simulink library "lib_Convection_TubeBankZukauskas"  (R2015a)
settings: Solver=ode45  StartTime=0.0  StopTime=10.0  RelTol=1e-3
libraries: simulink x24, lib_GenTools_MinMax x1
settings Model: Creator=jlkratz  LastModifiedBy=jlkratz

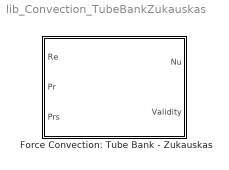
== system lib_Convection_TubeBankZukauskas ==
  Force Convection: Tube Bank - Zukauskas : Subsystem  mask(TSAT: Tube Bank - Zukauskas){N_M=20, StSLratio_M=4, AlignOrStag_M=on}
      mask prompts: N_M "N_M - Number of rows of tubes"; StSLratio_M "StSLratio_M - Ratio of distances between tubes in the transverse direction and flow direction (St/SL)"; AlignOrStag_M "AlignOrStag_M - Checked for aligned tubes and unchecked for staggered tubes"
      mask help:
      | This block estimates the average Nusselt number for an entire bank of cylinderical tubes using a correlation proposed by Zukauskas. The tube bank may consist of rows of tubes that are aligned with each other or staggered. The Reynolds number (Re) should be calculated based on the diameter of the largest cylinder in the bank. The properties of the fluid should be evaluated at the mean of the fluid inlet and outlet temperatures with the exception of Prs which is the Prantl number (Pr) evaluated using the temperature of the surface of the tubes. If the surface temperature of each tube differs then a rough approximation could be possible by using the average surface temperature of all the tubes. The correlation is best suited for banks with 20 or more rows of tubes but this implemenation does consider adjustments for banks with less than 20 rows. The correlation is subject to the following restricitons:
      |
      | 10 <= Re <= 2000000
      | 0.7 <= Pr <= 500
      |
      | For additional information see the block help menu.
      mask Help: web(which('Convection_TSAT_TubeBankZukauskus.html'),'-helpbrowser')
      mask DialogControl Container3 Prompt: Parameters

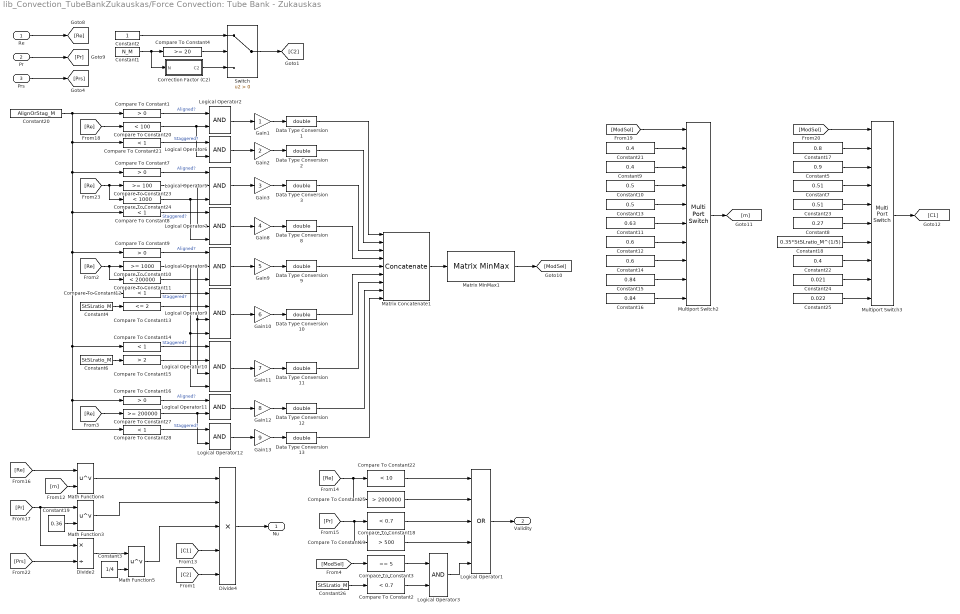
== system lib_Convection_TubeBankZukauskas/Force Convection: Tube Bank - Zukauskas ==
  Re : Inport
  Pr : Inport  Port=2
  Prs : Inport  Port=3
  Compare To Constant{1,7,9,16} (4 alike) : simulink/Logic and Bit Operations/Compare To Constant  relop=>  const=0  OutDataTypeStr=boolean
  Compare To Constant10 : simulink/Logic and Bit Operations/Compare To Constant  relop=>=  const=1000  OutDataTypeStr=boolean
  Compare To Constant11 : simulink/Logic and Bit Operations/Compare To Constant  relop=<  const=200000  OutDataTypeStr=boolean
  Compare To Constant{8,12,14,21,28} (5 alike) : simulink/Logic and Bit Operations/Compare To Constant  relop=<  const=1  OutDataTypeStr=boolean
  Compare To Constant13 : simulink/Logic and Bit Operations/Compare To Constant  relop=<=  const=2  OutDataTypeStr=boolean
  Compare To Constant15 : simulink/Logic and Bit Operations/Compare To Constant  relop=>  const=2  OutDataTypeStr=boolean
  Compare To Constant18 : simulink/Logic and Bit Operations/Compare To Constant  relop=<  const=0.7  OutDataTypeStr=boolean
  Compare To Constant19 : simulink/Logic and Bit Operations/Compare To Constant  relop=>  const=500  OutDataTypeStr=boolean
  Compare To Constant2 : simulink/Logic and Bit Operations/Compare To Constant  relop=<  const=0.7  OutDataTypeStr=boolean
  Compare To Constant20 : simulink/Logic and Bit Operations/Compare To Constant  relop=<  const=100  OutDataTypeStr=boolean
  Compare To Constant22 : simulink/Logic and Bit Operations/Compare To Constant  relop=<  const=10  OutDataTypeStr=boolean
  Compare To Constant23 : simulink/Logic and Bit Operations/Compare To Constant  relop=>=  const=100  OutDataTypeStr=boolean
  Compare To Constant24 : simulink/Logic and Bit Operations/Compare To Constant  relop=<  const=1000  OutDataTypeStr=boolean
  Compare To Constant25 : simulink/Logic and Bit Operations/Compare To Constant  relop=>  const=2000000  OutDataTypeStr=boolean
  Compare To Constant27 : simulink/Logic and Bit Operations/Compare To Constant  relop=>=  const=200000  OutDataTypeStr=boolean
  Compare To Constant3 : simulink/Logic and Bit Operations/Compare To Constant  relop===  const=5  OutDataTypeStr=boolean
  Compare To Constant4 : simulink/Logic and Bit Operations/Compare To Constant  relop=>=  const=20  OutDataTypeStr=boolean
  Constant1 : Constant  Value=N_M
  Constant10 : Constant  Value=0.5
  Constant11 : Constant  Value=0.63
  Constant12 : Constant  Value=0.6
  Constant13 : Constant  Value=0.5
  Constant14 : Constant  Value=0.6
  Constant15 : Constant  Value=0.84
  Constant16 : Constant  Value=0.84
  Constant17 : Constant  Value=0.8
  Constant18 : Constant  Value=0.35*StSLratio_M^(1/5)
  Constant19 : Constant  Value=0.36
  Constant2 : Constant
  Constant20 : Constant  Value=AlignOrStag_M
  Constant21 : Constant  Value=0.4
  Constant22 : Constant  Value=0.4
  Constant23 : Constant  Value=0.51
  Constant24 : Constant  Value=0.021
  Constant25 : Constant  Value=0.022
  Constant26 : Constant  Value=StSLratio_M
  Constant3 : Constant  Value=1/4
  Constant4 : Constant  Value=StSLratio_M
  Constant5 : Constant  Value=0.9
  Constant6 : Constant  Value=StSLratio_M
  Constant7 : Constant  Value=0.51
  Constant8 : Constant  Value=0.27
  Constant9 : Constant  Value=0.4
  Correction Factor (C2) : Subsystem
  Data Type Conversion{1..3,8..13} (9 alike) : DataTypeConversion  OutDataTypeStr=double
  Divide2 : Product  Inputs=*/
  Divide4 : Product  Inputs=*****
  Gain1 : Gain
  Gain10 : Gain  Gain=6
  Gain11 : Gain  Gain=7
  Gain12 : Gain  Gain=8
  Gain13 : Gain  Gain=9
  Gain2 : Gain  Gain=2
  Gain3 : Gain  Gain=3
  Gain8 : Gain  Gain=4
  Gain9 : Gain  Gain=5
  Logical Operator1 : Logic  Operator=OR  Inputs=5  AllPortsSameDT=off  OutDataTypeStr=boolean
  Logical Operator10 : Logic  Inputs=4  AllPortsSameDT=off  OutDataTypeStr=boolean
  Logical Operator{2..3,6,11..12} (5 alike) : Logic  AllPortsSameDT=off  OutDataTypeStr=boolean
  Logical Operator5 : Logic  Inputs=3  AllPortsSameDT=off  OutDataTypeStr=boolean
  Logical Operator7 : Logic  Inputs=3  AllPortsSameDT=off  OutDataTypeStr=boolean
  Logical Operator8 : Logic  Inputs=3  AllPortsSameDT=off  OutDataTypeStr=boolean
  Logical Operator9 : Logic  Inputs=4  AllPortsSameDT=off  OutDataTypeStr=boolean
  Math Function3 : Math  Operator=pow  SaturateOnIntegerOverflow=on
  Math Function4 : Math  Operator=pow  SaturateOnIntegerOverflow=on
  Math Function5 : Math  Operator=pow  SaturateOnIntegerOverflow=on
  Matrix Concatenate1 : Concatenate  NumInputs=9  Mode=Multidimensional array  ConcatenateDimension=2
  Matrix MinMax1 : lib_GenTools_MinMax/Matrix MinMax  rows_M=on  cols_M=off  all_M=off  minmax_M=off  BN_M=gcb
  Multiport Switch2 : MultiPortSwitch  Inputs=9
  Multiport Switch3 : MultiPortSwitch  Inputs=9
  Switch : Switch  Criteria=u2 > Threshold
  Nu : Outport
  Validity : Outport  Port=2
  wires:
  Logical Operator3/1 -> Logical Operator1/5
  Compare To Constant2/1 -> Logical Operator3/2
  Compare To Constant3/1 -> Logical Operator3/1
  [ModSel] -> Compare To Constant3/1
  Constant26/1 -> Compare To Constant2/1
  Logical Operator1/1 -> Validity/1
  Constant22/1 -> Multiport Switch3/8
  Constant18/1 -> Multiport Switch3/7
  Constant8/1 -> Multiport Switch3/6
  Constant23/1 -> Multiport Switch3/5
  Constant25/1 -> Multiport Switch3/10
  Constant24/1 -> Multiport Switch3/9
  Constant16/1 -> Multiport Switch2/10
  Constant15/1 -> Multiport Switch2/9
  Constant14/1 -> Multiport Switch2/8
  Constant12/1 -> Multiport Switch2/7
  Constant11/1 -> Multiport Switch2/6
  Data Type Conversion13/1 -> Matrix Concatenate1/9
  Data Type Conversion12/1 -> Matrix Concatenate1/8
  Data Type Conversion11/1 -> Matrix Concatenate1/7
  Data Type Conversion10/1 -> Matrix Concatenate1/6
  Data Type Conversion9/1 -> Matrix Concatenate1/5
  Data Type Conversion8/1 -> Matrix Concatenate1/4
  Data Type Conversion3/1 -> Matrix Concatenate1/3
  Data Type Conversion2/1 -> Matrix Concatenate1/2
  Data Type Conversion1/1 -> Matrix Concatenate1/1
  Logical Operator12/1 -> Gain13/1
  Logical Operator11/1 -> Gain12/1
  Gain13/1 -> Data Type Conversion13/1
  Gain12/1 -> Data Type Conversion12/1
  Compare To Constant28/1 -> Logical Operator12/1  "Staggered?"
  Compare To Constant27/1 -> Logical Operator11/2, Logical Operator12/2
  Compare To Constant16/1 -> Logical Operator11/1  "Aligned?"
  [Re] -> Compare To Constant27/1
  Logical Operator10/1 -> Gain11/1
  Logical Operator9/1 -> Gain10/1
  Logical Operator8/1 -> Gain9/1
  Gain11/1 -> Data Type Conversion11/1
  Gain10/1 -> Data Type Conversion10/1
  Gain9/1 -> Data Type Conversion9/1
  Compare To Constant15/1 -> Logical Operator10/2
  Constant6/1 -> Compare To Constant15/1
  Compare To Constant14/1 -> Logical Operator10/1  "Staggered?"
  Compare To Constant13/1 -> Logical Operator9/2
  Compare To Constant12/1 -> Logical Operator9/1  "Staggered?"
  Constant4/1 -> Compare To Constant13/1
  Compare To Constant11/1 -> Logical Operator8/3
  Compare To Constant10/1 -> Logical Operator8/2, Logical Operator10/3, Logical Operator9/3, Logical Operator9/4, Logical Operator10/4
  Compare To Constant9/1 -> Logical Operator8/1  "Aligned?"
  [Re] -> Compare To Constant11/1, Compare To Constant10/1
  Logical Operator7/1 -> Gain8/1
  Gain8/1 -> Data Type Conversion8/1
  Compare To Constant8/1 -> Logical Operator7/1  "Staggered?"
  Constant20/1 -> Compare To Constant1/1, Compare To Constant21/1, Compare To Constant7/1, Compare To Constant9/1, Compare To Constant12/1, Compare To Constant14/1, Compare To Constant28/1, Compare To Constant16/1, Compare To Constant8/1
  Logical Operator5/1 -> Gain3/1
  Gain3/1 -> Data Type Conversion3/1
  Compare To Constant24/1 -> Logical Operator5/3, Logical Operator7/3
  Compare To Constant23/1 -> Logical Operator5/2, Logical Operator7/2
  Compare To Constant7/1 -> Logical Operator5/1  "Aligned?"
  Logical Operator6/1 -> Gain2/1
  Gain2/1 -> Data Type Conversion2/1
  Logical Operator2/1 -> Gain1/1
  Gain1/1 -> Data Type Conversion1/1
  Compare To Constant21/1 -> Logical Operator6/1  "Staggered?"
  Correction Factor (C2)/1(C2) -> Switch/3
  Constant2/1 -> Switch/1
  [C2] -> Divide4/5
  Switch/1 -> [C2]
  Compare To Constant4/1 -> Switch/2
  Constant1/1 -> Compare To Constant4/1, Correction Factor (C2)/1(N)
  [Re] -> Compare To Constant23/1, Compare To Constant24/1
  Compare To Constant20/1 -> Logical Operator2/2, Logical Operator6/2
  [Re] -> Compare To Constant20/1
  Compare To Constant1/1 -> Logical Operator2/1  "Aligned?"
  Compare To Constant19/1 -> Logical Operator1/4
  Compare To Constant18/1 -> Logical Operator1/3
  Compare To Constant25/1 -> Logical Operator1/2
  Compare To Constant22/1 -> Logical Operator1/1
  [Pr] -> Compare To Constant18/1, Compare To Constant19/1
  [Re] -> Compare To Constant22/1, Compare To Constant25/1
  Math Function5/1 -> Divide4/3
  Math Function3/1 -> Divide4/2
  Math Function4/1 -> Divide4/1
  [C1] -> Divide4/4
  Constant3/1 -> Math Function5/2
  Divide2/1 -> Math Function5/1
  [Prs] -> Divide2/2
  [Pr] -> Math Function3/1, Divide2/1
  [Re] -> Math Function4/1
  Prs/1 -> [Prs]
  Matrix Concatenate1/1 -> Matrix MinMax1/1
  Matrix MinMax1/1 -> [ModSel]
  Constant7/1 -> Multiport Switch3/4
  Constant5/1 -> Multiport Switch3/3
  Constant17/1 -> Multiport Switch3/2
  Constant13/1 -> Multiport Switch2/5
  Constant10/1 -> Multiport Switch2/4
  Constant9/1 -> Multiport Switch2/3
  Constant21/1 -> Multiport Switch2/2
  Multiport Switch3/1 -> [C1]
  Multiport Switch2/1 -> [m]
  [ModSel] -> Multiport Switch3/1
  [ModSel] -> Multiport Switch2/1
  Pr/1 -> [Pr]
  Re/1 -> [Re]
  Divide4/1 -> Nu/1
  [m] -> Math Function4/2
  Constant19/1 -> Math Function3/2

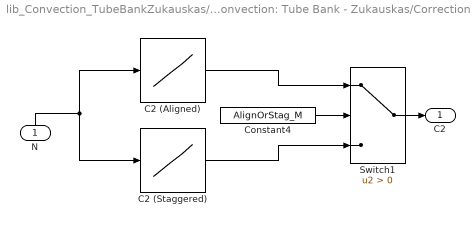
== system lib_Convection_TubeBankZukauskas/Force Convection: Tube Bank - Zukauskas/Correction Factor (C2) ==
  N : Inport
  C2 (Aligned) : Lookup_n-D  NumberOfTableDimensions=1  BreakpointsForDimension1=[1 2 3 4 5 7 10 13 16 20]  Table=[0.7 0.8 0.86 0.9 0.92 0.95 0.97 0.98 0.99 1]  InternalRulePriority=Speed  RndMeth=Simplest  InputSameDT=on
  C2 (Staggered) : Lookup_n-D  NumberOfTableDimensions=1  BreakpointsForDimension1=[1 2 3 4 5 7 10 13 16 20]  Table=[0.64 0.76 0.84 0.89 0.92 0.95 0.97 0.98 0.99 1]  InternalRulePriority=Speed  RndMeth=Simplest  InputSameDT=on
  Constant4 : Constant  Value=AlignOrStag_M
  Switch1 : Switch  Criteria=u2 > Threshold
  C2 : Outport
  wires:
  Constant4/1 -> Switch1/2
  C2 (Aligned)/1 -> Switch1/1
  N/1 -> C2 (Staggered)/1, C2 (Aligned)/1
  C2 (Staggered)/1 -> Switch1/3
  Switch1/1 -> C2/1
